simulink subsystem "Weighted_Sum_Avg_No_ABF"  (R2020b)
settings: Solver=VariableStepAuto  StartTime=0.0  StopTime=10.0  RelTol=1e-3
values from neighbouring files (symbols this model uses):
  N = 8    [env_sim_setup.m]
settings Model: Creator=jgentile  LastModifiedBy=jgentile

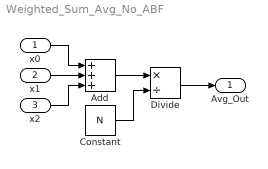
== system Weighted_Sum_Avg_No_ABF ==
  x0 : Inport
  x1 : Inport  Port=2
  x2 : Inport  Port=3
  Add : Sum  Inputs=+++
  Constant : Constant  Value=N
  Divide : Product  Inputs=*/
  Avg_Out : Outport
  wires:
  x0/1 -> Add/1
  x2/1 -> Add/3
  Constant/1 -> Divide/2
  Add/1 -> Divide/1
  x1/1 -> Add/2
  Divide/1 -> Avg_Out/1
